simulink model "quat_prop_hrn"  (R2014b)
settings: Solver=ode45  StartTime=0.0  StopTime=20  FixedStep=0.1  MaxStep=0.1  RelTol=1e-3
values from neighbouring files (symbols this model uses):
  dt = 0.1    [quat_prop_test.m]
libraries: util_quat_lib x1
settings Model: Creator=Administrator  LastModifiedBy=mstewart
settings DataIOCC: SignalLoggingSaveFormat=ModelDataLogs
settings OptimizationCC: ExpressionDepthLimit=2147483647  InitFltsAndDblsToZero=on
settings DebuggingCC: UnderspecifiedInitializationDetection=Classic  MergeDetectMultiDrivingBlocksExec=none  FcnCallInpInsideContextMsg=UseLocalSettings  StateNameClashWarn=warning  StrictBusMsg=Warning
settings GRTTargetCC: CombineOutputUpdateFcns=off  GRTInterface=on

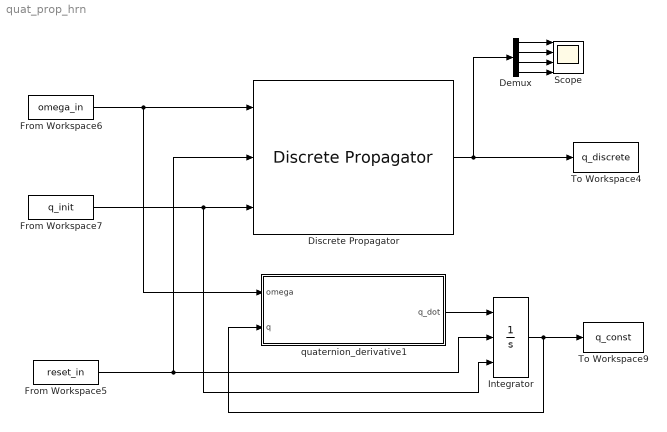
== system quat_prop_hrn ==
  Demux : Demux
  Discrete Propagator : util_quat_lib/Discrete Propagator  SystemSampleTime=dt
  From Workspace5 : FromWorkspace  VariableName=reset_in  SampleTime=dt  Interpolate=off  OutputAfterFinalValue=Setting to zero
  From Workspace6 : FromWorkspace  VariableName=omega_in  SampleTime=dt  Interpolate=off  OutputAfterFinalValue=Setting to zero
  From Workspace7 : FromWorkspace  VariableName=q_init  SampleTime=0
  Integrator : Integrator  ExternalReset=rising  InitialConditionSource=external  InitialCondition=[0 0 0 1]
  Scope : Scope  NumInputPorts=4
      settings: YMin=-1~-1~-1~0.95  YMax=1~1~1~1.05
  To Workspace4 : ToWorkspace  VariableName=q_discrete  SampleTime=-1
  To Workspace9 : ToWorkspace  VariableName=q_const  SaveFormat=Structure With Time  SampleTime=-1
  quaternion_derivative1 : Subsystem
      mask Display: disp('d/dt(q)')
  wires:
  quaternion_derivative1/1(q_dot) -> Integrator/1
  Integrator/1 -> quaternion_derivative1/2(q), To Workspace9/1
  From Workspace7/1 -> Integrator/3, Discrete Propagator/3
  From Workspace6/1 -> quaternion_derivative1/1(omega), Discrete Propagator/1
  From Workspace5/1 -> Integrator/2, Discrete Propagator/2
  Demux/1 -> Scope/1
  Demux/2 -> Scope/2
  Demux/3 -> Scope/3
  Demux/4 -> Scope/4
  Discrete Propagator/1 -> To Workspace4/1, Demux/1

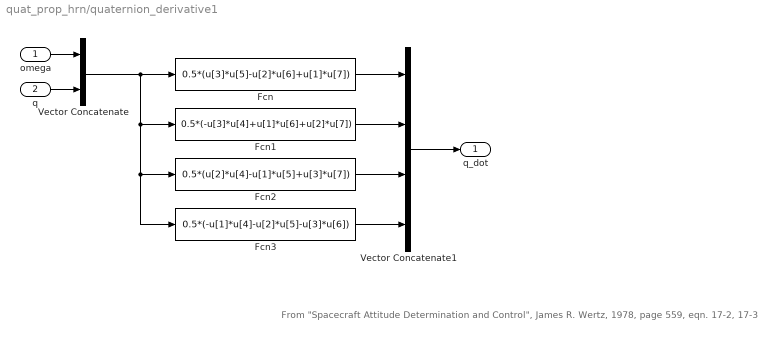
== system quat_prop_hrn/quaternion_derivative1 ==
  note: From "Spacecraft Attitude Determination and Control", James R. Wertz, 1978, page 559, eqn. 17-2, 17-3
  omega : Inport
  q : Inport  Port=2
  Fcn : Fcn  Expr=0.5*(u[3]*u[5]-u[2]*u[6]+u[1]*u[7])
  Fcn1 : Fcn  Expr=0.5*(-u[3]*u[4]+u[1]*u[6]+u[2]*u[7])
  Fcn2 : Fcn  Expr=0.5*(u[2]*u[4]-u[1]*u[5]+u[3]*u[7])
  Fcn3 : Fcn  Expr=0.5*(-u[1]*u[4]-u[2]*u[5]-u[3]*u[6])
  Vector Concatenate : Concatenate
  Vector Concatenate1 : Concatenate  NumInputs=4
  q_dot : Outport
  wires:
  Vector Concatenate/1 -> Fcn/1, Fcn1/1, Fcn2/1, Fcn3/1
  Fcn3/1 -> Vector Concatenate1/4
  Fcn/1 -> Vector Concatenate1/1
  Fcn1/1 -> Vector Concatenate1/2
  Fcn2/1 -> Vector Concatenate1/3
  omega/1 -> Vector Concatenate/1
  q/1 -> Vector Concatenate/2
  Vector Concatenate1/1 -> q_dot/1
